simulink model "simpleMicrogrid_PhasorEMT"  (R2017b)
settings: Solver=ode23tb  StartTime=0.0  StopTime=60  RelTol=1e-3
InitFcn:
  | Ts = 1e-4;
  | Rs = 4;
  | Ls = 0;
  | kv = 1;
undefined symbols (not defined in the file): DiscIntNeverNeededParam, Tlim
libraries: powerlib x65, powerlib_meascontrol x7, simulink x6, sps_avr x1, spsDieselMotorModel x1
(part 2 of 2)

== system simpleMicrogrid_PhasorEMT/Electromagnetic Transient/SPS-Simulink Interface/Phasor/Vc ==
  Vin : Inport
  Controlled Voltage Source : powerlib/Electrical Sources/Controlled Voltage Source  Initialize=off  Source_Type=AC  Amplitude=0  Phase=0  Frequency=0  Measurements=None
  Gain : Gain  Gain=kv
  Series RLC Branch : powerlib/Elements/Series RLC Branch  LConnTagsString=__new0  RConnTagsString=__new0  BranchType=R  Resistance=Rs  Inductance=1e-3  SetiL0=off  InitialCurrent=0  Capacitance=1e-6  Setx0=off  InitialVoltage=0  Measurements=None
  Sum : Sum
  Voltage Measurement : powerlib/Measurements/Voltage Measurement  PhasorSimulation=off  OutputType=Complex  PSBequivalent=0
  Voltage Measurement1 : powerlib/Measurements/Voltage Measurement  PhasorSimulation=off  OutputType=Complex  PSBequivalent=0
  + : PMIOPort  Port=1  Side=Left
  - : PMIOPort  Port=2  Side=Right
  Vout : Outport
  wires:
  Gain/1 -> Sum/1
  Voltage Measurement/1 -> Sum/2
  Voltage Measurement1/1 -> Gain/1
  Vin/1 -> Controlled Voltage Source/1
  Sum/1 -> Vout/1
  connections:
  Voltage Measurement/LConn2 -- -/RConn1 -- Controlled Voltage Source/LConn1
  Voltage Measurement1/LConn1 -- Voltage Measurement/LConn1 -- Series RLC Branch/LConn1 -- +/RConn1
  Controlled Voltage Source/RConn1 -- Voltage Measurement1/LConn2 -- Series RLC Branch/RConn1

== system simpleMicrogrid_PhasorEMT/Phasor/SPS-Simulink Interface/EMT/Frequency Generator ==
  Continuous : Subsystem  VariantControl=Continuous
  Discrete : Subsystem  VariantControl=Discrete
  2pi*f : Outport

== system simpleMicrogrid_PhasorEMT/Phasor/SPS-Simulink Interface/EMT/Va ==
  Vin : Inport
  Controlled Voltage Source : powerlib/Electrical Sources/Controlled Voltage Source  Initialize=off  Source_Type=AC  Amplitude=0  Phase=0  Frequency=0  Measurements=None
  Gain : Gain  Gain=kv
  Series RLC Branch : powerlib/Elements/Series RLC Branch  LConnTagsString=__new0  RConnTagsString=__new0  BranchType=RL  Resistance=Rs  Inductance=Ls  SetiL0=off  InitialCurrent=0  Capacitance=1e-6  Setx0=off  InitialVoltage=0  Measurements=None
  Sum : Sum
  Voltage Measurement : powerlib/Measurements/Voltage Measurement  PhasorSimulation=on  OutputType=Complex  PSBequivalent=0
  Voltage Measurement1 : powerlib/Measurements/Voltage Measurement  PhasorSimulation=on  OutputType=Complex  PSBequivalent=0
  + : PMIOPort  Port=1  Side=Left
  - : PMIOPort  Port=2  Side=Right
  Vout : Outport
  wires:
  Voltage Measurement/1 -> Sum/2
  Voltage Measurement1/1 -> Gain/1
  Vin/1 -> Controlled Voltage Source/1
  Sum/1 -> Vout/1
  Gain/1 -> Sum/1
  connections:
  Voltage Measurement/LConn2 -- -/RConn1 -- Controlled Voltage Source/LConn1
  Voltage Measurement1/LConn1 -- Voltage Measurement/LConn1 -- Series RLC Branch/LConn1 -- +/RConn1
  Controlled Voltage Source/RConn1 -- Voltage Measurement1/LConn2 -- Series RLC Branch/RConn1

== system simpleMicrogrid_PhasorEMT/Phasor/SPS-Simulink Interface/EMT/Va1 ==
  Vin : Inport
  Controlled Voltage Source : powerlib/Electrical Sources/Controlled Voltage Source  Initialize=off  Source_Type=AC  Amplitude=0  Phase=0  Frequency=0  Measurements=None
  Gain : Gain  Gain=kv
  Series RLC Branch : powerlib/Elements/Series RLC Branch  LConnTagsString=__new0  RConnTagsString=__new0  BranchType=RL  Resistance=Rs  Inductance=Ls  SetiL0=off  InitialCurrent=0  Capacitance=1e-6  Setx0=off  InitialVoltage=0  Measurements=None
  Sum : Sum
  Voltage Measurement : powerlib/Measurements/Voltage Measurement  PhasorSimulation=on  OutputType=Complex  PSBequivalent=0
  Voltage Measurement1 : powerlib/Measurements/Voltage Measurement  PhasorSimulation=on  OutputType=Complex  PSBequivalent=0
  + : PMIOPort  Port=1  Side=Left
  - : PMIOPort  Port=2  Side=Right
  Vout : Outport
  wires:
  Gain/1 -> Sum/1
  Sum/1 -> Vout/1
  Vin/1 -> Controlled Voltage Source/1
  Voltage Measurement1/1 -> Gain/1
  Voltage Measurement/1 -> Sum/2
  connections:
  Series RLC Branch/RConn1 -- Voltage Measurement1/LConn2 -- Controlled Voltage Source/RConn1
  +/RConn1 -- Series RLC Branch/LConn1 -- Voltage Measurement/LConn1 -- Voltage Measurement1/LConn1
  Controlled Voltage Source/LConn1 -- -/RConn1 -- Voltage Measurement/LConn2

== system simpleMicrogrid_PhasorEMT/Phasor/SPS-Simulink Interface/EMT/Va2 ==
  Vin : Inport
  Controlled Voltage Source : powerlib/Electrical Sources/Controlled Voltage Source  Initialize=off  Source_Type=AC  Amplitude=0  Phase=0  Frequency=0  Measurements=None
  Gain : Gain  Gain=kv
  Series RLC Branch : powerlib/Elements/Series RLC Branch  LConnTagsString=__new0  RConnTagsString=__new0  BranchType=RL  Resistance=Rs  Inductance=Ls  SetiL0=off  InitialCurrent=0  Capacitance=1e-6  Setx0=off  InitialVoltage=0  Measurements=None
  Sum : Sum
  Voltage Measurement : powerlib/Measurements/Voltage Measurement  PhasorSimulation=on  OutputType=Complex  PSBequivalent=0
  Voltage Measurement1 : powerlib/Measurements/Voltage Measurement  PhasorSimulation=on  OutputType=Complex  PSBequivalent=0
  + : PMIOPort  Port=1  Side=Left
  - : PMIOPort  Port=2  Side=Right
  Vout : Outport
  wires:
  Voltage Measurement/1 -> Sum/2
  Voltage Measurement1/1 -> Gain/1
  Vin/1 -> Controlled Voltage Source/1
  Sum/1 -> Vout/1
  Gain/1 -> Sum/1
  connections:
  Voltage Measurement/LConn2 -- -/RConn1 -- Controlled Voltage Source/LConn1
  Voltage Measurement1/LConn1 -- Voltage Measurement/LConn1 -- Series RLC Branch/LConn1 -- +/RConn1
  Controlled Voltage Source/RConn1 -- Voltage Measurement1/LConn2 -- Series RLC Branch/RConn1

== system simpleMicrogrid_PhasorEMT/Phasor/SPS-Simulink Interface/Phasor/Va ==
  Vin : Inport
  Controlled Voltage Source : powerlib/Electrical Sources/Controlled Voltage Source  Initialize=off  Source_Type=AC  Amplitude=0  Phase=0  Frequency=0  Measurements=None
  Gain : Gain  Gain=kv
  Series RLC Branch : powerlib/Elements/Series RLC Branch  LConnTagsString=__new0  RConnTagsString=__new0  BranchType=R  Resistance=Rs  Inductance=1e-3  SetiL0=off  InitialCurrent=0  Capacitance=1e-6  Setx0=off  InitialVoltage=0  Measurements=None
  Sum : Sum
  Voltage Measurement : powerlib/Measurements/Voltage Measurement  PhasorSimulation=on  OutputType=Complex  PSBequivalent=0
  Voltage Measurement1 : powerlib/Measurements/Voltage Measurement  PhasorSimulation=on  OutputType=Complex  PSBequivalent=0
  + : PMIOPort  Port=1  Side=Left
  - : PMIOPort  Port=2  Side=Right
  Vout : Outport
  wires:
  Gain/1 -> Sum/1
  Voltage Measurement/1 -> Sum/2
  Voltage Measurement1/1 -> Gain/1
  Vin/1 -> Controlled Voltage Source/1
  Sum/1 -> Vout/1
  connections:
  Voltage Measurement/LConn2 -- -/RConn1 -- Controlled Voltage Source/LConn1
  Voltage Measurement1/LConn1 -- Voltage Measurement/LConn1 -- Series RLC Branch/LConn1 -- +/RConn1
  Controlled Voltage Source/RConn1 -- Voltage Measurement1/LConn2 -- Series RLC Branch/RConn1

== system simpleMicrogrid_PhasorEMT/Phasor/SPS-Simulink Interface/Phasor/Vb ==
  Vin : Inport
  Controlled Voltage Source : powerlib/Electrical Sources/Controlled Voltage Source  Initialize=off  Source_Type=AC  Amplitude=0  Phase=0  Frequency=0  Measurements=None
  Gain : Gain  Gain=kv
  Series RLC Branch : powerlib/Elements/Series RLC Branch  LConnTagsString=__new0  RConnTagsString=__new0  BranchType=R  Resistance=Rs  Inductance=1e-3  SetiL0=off  InitialCurrent=0  Capacitance=1e-6  Setx0=off  InitialVoltage=0  Measurements=None
  Sum : Sum
  Voltage Measurement : powerlib/Measurements/Voltage Measurement  PhasorSimulation=on  OutputType=Complex  PSBequivalent=0
  Voltage Measurement1 : powerlib/Measurements/Voltage Measurement  PhasorSimulation=on  OutputType=Complex  PSBequivalent=0
  + : PMIOPort  Port=1  Side=Left
  - : PMIOPort  Port=2  Side=Right
  Vout : Outport
  wires:
  Sum/1 -> Vout/1
  Vin/1 -> Controlled Voltage Source/1
  Voltage Measurement1/1 -> Gain/1
  Voltage Measurement/1 -> Sum/2
  Gain/1 -> Sum/1
  connections:
  Series RLC Branch/RConn1 -- Voltage Measurement1/LConn2 -- Controlled Voltage Source/RConn1
  +/RConn1 -- Series RLC Branch/LConn1 -- Voltage Measurement/LConn1 -- Voltage Measurement1/LConn1
  Controlled Voltage Source/LConn1 -- -/RConn1 -- Voltage Measurement/LConn2

== system simpleMicrogrid_PhasorEMT/Phasor/SPS-Simulink Interface/Phasor/Vc ==
  Vin : Inport
  Controlled Voltage Source : powerlib/Electrical Sources/Controlled Voltage Source  Initialize=off  Source_Type=AC  Amplitude=0  Phase=0  Frequency=0  Measurements=None
  Gain : Gain  Gain=kv
  Series RLC Branch : powerlib/Elements/Series RLC Branch  LConnTagsString=__new0  RConnTagsString=__new0  BranchType=R  Resistance=Rs  Inductance=1e-3  SetiL0=off  InitialCurrent=0  Capacitance=1e-6  Setx0=off  InitialVoltage=0  Measurements=None
  Sum : Sum
  Voltage Measurement : powerlib/Measurements/Voltage Measurement  PhasorSimulation=on  OutputType=Complex  PSBequivalent=0
  Voltage Measurement1 : powerlib/Measurements/Voltage Measurement  PhasorSimulation=on  OutputType=Complex  PSBequivalent=0
  + : PMIOPort  Port=1  Side=Left
  - : PMIOPort  Port=2  Side=Right
  Vout : Outport
  wires:
  Gain/1 -> Sum/1
  Voltage Measurement/1 -> Sum/2
  Voltage Measurement1/1 -> Gain/1
  Vin/1 -> Controlled Voltage Source/1
  Sum/1 -> Vout/1
  connections:
  Voltage Measurement/LConn2 -- -/RConn1 -- Controlled Voltage Source/LConn1
  Voltage Measurement1/LConn1 -- Voltage Measurement/LConn1 -- Series RLC Branch/LConn1 -- +/RConn1
  Controlled Voltage Source/RConn1 -- Voltage Measurement1/LConn2 -- Series RLC Branch/RConn1

== system simpleMicrogrid_PhasorEMT/Electromagnetic Transient/SPS-Simulink Interface/EMT/Frequency Generator/Continuous ==
  Clock : Clock
  Constant4 : Constant  Value=2*pi
  Freq1 : Constant  Value=Freq
  Freq2 : Constant  Value=2*pi
  Math Function : Math  Operator=mod  SaturateOnIntegerOverflow=on
  Product3 : Product  Inputs=***  SaturateOnIntegerOverflow=on  InputSameDT=on  OutDataTypeStr=Inherit: Same as first input
  2pi*f : Outport
  wires:
  Clock/1 -> Product3/2
  Freq2/1 -> Product3/3
  Freq1/1 -> Product3/1
  Constant4/1 -> Math Function/2
  Product3/1 -> Math Function/1
  Math Function/1 -> 2pi*f/1

== system simpleMicrogrid_PhasorEMT/Electromagnetic Transient/SPS-Simulink Interface/EMT/Frequency Generator/Discrete ==
  Constant4 : Constant  Value=2*pi
  Freq1 : Constant  Value=Freq
  Freq2 : Constant  Value=2*pi
  Math Function : Math  Operator=mod  SaturateOnIntegerOverflow=on
  Product3 : Product  Inputs=***  SaturateOnIntegerOverflow=on  InputSameDT=on  OutDataTypeStr=Inherit: Same as first input
  t : DigitalClock  SampleTime=Ts
  2pi*f : Outport
  wires:
  Math Function/1 -> 2pi*f/1
  Product3/1 -> Math Function/1
  Constant4/1 -> Math Function/2
  Freq1/1 -> Product3/1
  Freq2/1 -> Product3/3
  t/1 -> Product3/2

== system simpleMicrogrid_PhasorEMT/Phasor/SPS-Simulink Interface/EMT/Frequency Generator/Continuous ==
  Clock : Clock
  Constant4 : Constant  Value=2*pi
  Freq1 : Constant  Value=Freq
  Freq2 : Constant  Value=2*pi
  Math Function : Math  Operator=mod  SaturateOnIntegerOverflow=on
  Product3 : Product  Inputs=***  SaturateOnIntegerOverflow=on  InputSameDT=on  OutDataTypeStr=Inherit: Same as first input
  2pi*f : Outport
  wires:
  Clock/1 -> Product3/2
  Freq2/1 -> Product3/3
  Freq1/1 -> Product3/1
  Constant4/1 -> Math Function/2
  Product3/1 -> Math Function/1
  Math Function/1 -> 2pi*f/1

== system simpleMicrogrid_PhasorEMT/Phasor/SPS-Simulink Interface/EMT/Frequency Generator/Discrete ==
  Constant4 : Constant  Value=2*pi
  Freq1 : Constant  Value=Freq
  Freq2 : Constant  Value=2*pi
  Math Function : Math  Operator=mod  SaturateOnIntegerOverflow=on
  Product3 : Product  Inputs=***  SaturateOnIntegerOverflow=on  InputSameDT=on  OutDataTypeStr=Inherit: Same as first input
  t : DigitalClock  SampleTime=Ts
  2pi*f : Outport
  wires:
  Math Function/1 -> 2pi*f/1
  Product3/1 -> Math Function/1
  Constant4/1 -> Math Function/2
  Freq1/1 -> Product3/1
  Freq2/1 -> Product3/3
  t/1 -> Product3/2
